simulink model "SteadyCam"  (R2015b)
settings: Solver=FixedStepAuto  StartTime=0.0  StopTime=10.0  FixedStep=Ts  RelTol=1e-3
InitFcn:
  | InitSteady;
values from neighbouring files (symbols this model uses):
  GainGyro = 90/12000    (= 0.0075)    [InitSteady.m]
  InitTime = 2.9    [InitSteady.m]
  PID_Activator = 35    [InitSteady.m]
  Rad2Deg = 180/pi    (= 57.2957795131)    [InitSteady.m]
  Ts = 0.03    [InitSteady.m]
undefined symbols (not defined in the file or in its folder): DiscIntNeverNeededParam, HighValFilter, LowFilterVal
libraries: simulink x3, RASPlib x2
settings Model: Creator=Simón  LastModifiedBy=Simón

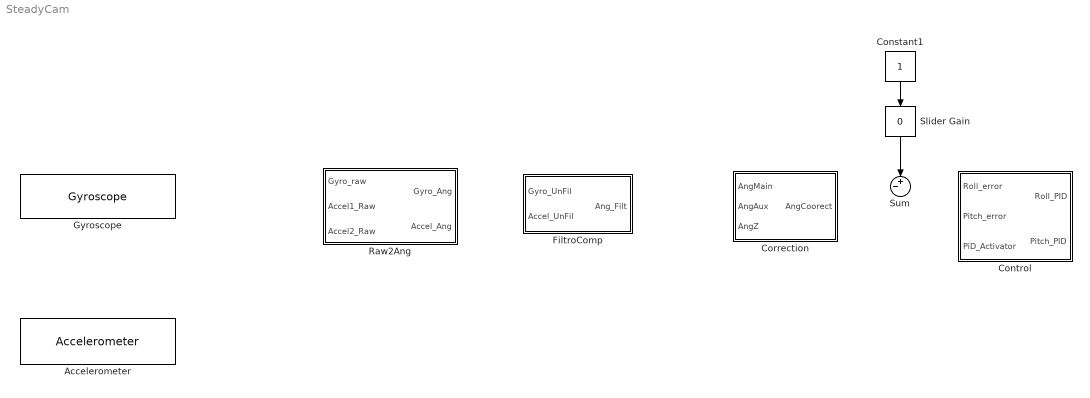
== system SteadyCam ==
  Accelerometer : RASPlib/Accelerometer  SimulateUsing=Code generation
  Constant1 : Constant
  Control : Subsystem
  Correction : Subsystem
  FiltroComp : Subsystem
  Gyroscope : RASPlib/Gyroscope  DLPFmode=0
  Raw2Ang : Subsystem
  Slider Gain : simulink/Math Operations/Slider Gain  low=-25  gain=0  high=35
  Sum : Sum  Inputs=+-|
  wires:
  Constant1/1 -> Slider Gain/1
  Slider Gain/1 -> Sum/1

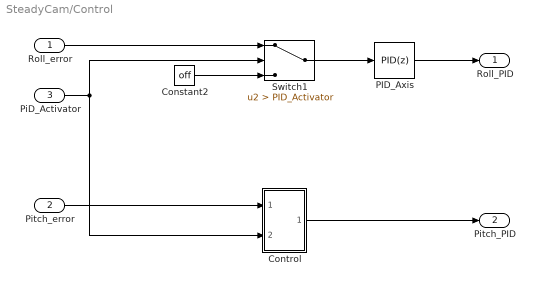
== system SteadyCam/Control ==
  Roll_error : Inport
  Pitch_error : Inport  Port=2
  PiD_Activator : Inport  Port=3
  Constant2 : Constant  Value=off
  Control : Subsystem
  PID_Axis : simulink/Continuous/PID Controller  Controller=PID  TimeDomain=Discrete-time  SampleTime=-1  IntegratorMethod=Forward Euler  FilterMethod=Forward Euler  Form=Parallel  UseFilter=off  ControllerParametersSource=internal  P=0.51  I=0.425  D=0.106  N=30  InitialConditionSource=internal  InitialConditionForIntegrator=0  InitialConditionForFilter=0  ExternalReset=none  LimitOutput=off  UpperSaturationLimit=inf  LowerSaturationLimit=-inf  LinearizeAsGain=off  AntiWindupMode=none  Kb=1  TrackingMode=off  Kt=1  PParamMin=[]  PParamMax=[]  IParamMin=[]  IParamMax=[]  DParamMin=[]  DParamMax=[]  NParamMin=[]  NParamMax=[]  KbParamMin=[]  KbParamMax=[]  KtParamMin=[]  KtParamMax=[]  POutMin=[]  POutMax=[]  IOutMin=[]  IOutMax=[]  DOutMin=[]  DOutMax=[]  NOutMin=[]  NOutMax=[]  KbOutMin=[]  KbOutMax=[]  KtOutMin=[]  KtOutMax=[]  IntegratorOutMin=[]  IntegratorOutMax=[]  FilterOutMin=[]  FilterOutMax=[]  SumOutMin=[]  SumOutMax=[]  SumI1OutMin=[]  SumI1OutMax=[]  SumI2OutMin=[]  SumI2OutMax=[]  SumI3OutMin=[]  SumI3OutMax=[]  SumDOutMin=[]  SumDOutMax=[]  SaturationOutMin=[]  SaturationOutMax=[]  IntegratorContinuousStateAttributes=''  IntegratorStateMustResolveToSignalObject=off  IntegratorRTWStateStorageClass=Auto  FilterContinuousStateAttributes=''  FilterStateMustResolveToSignalObject=off  FilterRTWStateStorageClass=Auto  DifferentiatorICPrevScaledInput=0  DifferentiatorOutMin=[]  DifferentiatorOutMax=[]
  Switch1 : Switch  Criteria=u2 > Threshold  Threshold=PID_Activator
  Roll_PID : Outport
  Pitch_PID : Outport  Port=2
  wires:
  Pitch_error/1 -> Control/1(In1)
  Control/1(Out1) -> Pitch_PID/1
  PID_Axis/1 -> Roll_PID/1
  Switch1/1 -> PID_Axis/1
  PiD_Activator/1 -> Switch1/2, Control/2(Threshold)
  Constant2/1 -> Switch1/3
  Roll_error/1 -> Switch1/1

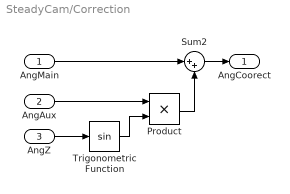
== system SteadyCam/Correction ==
  AngMain : Inport
  AngAux : Inport  Port=2
  AngZ : Inport  Port=3
  Product : Product
  Sum2 : Sum  Inputs=|++
  Trigonometric Function : Trigonometry
  AngCoorect : Outport
  wires:
  AngAux/1 -> Product/1
  Sum2/1 -> AngCoorect/1
  AngZ/1 -> Trigonometric Function/1
  AngMain/1 -> Sum2/1
  Product/1 -> Sum2/2
  Trigonometric Function/1 -> Product/2

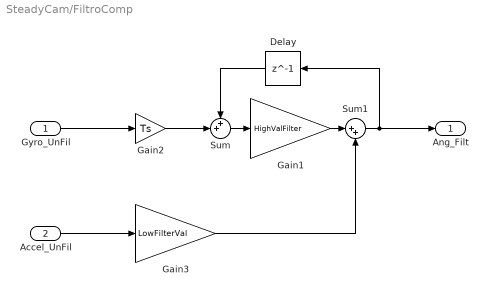
== system SteadyCam/FiltroComp ==
  Gyro_UnFil : Inport
  Accel_UnFil : Inport  Port=2
  Delay : Delay  DelayLength=1  InitialCondition=0
  Gain1 : Gain  Gain=HighValFilter
  Gain2 : Gain  Gain=Ts
  Gain3 : Gain  Gain=LowFilterVal
  Sum : Sum  Inputs=++|
  Sum1 : Sum  Inputs=|++
  Ang_Filt : Outport
  wires:
  Gain3/1 -> Sum1/2
  Gyro_UnFil/1 -> Gain2/1
  Sum1/1 -> Ang_Filt/1, Delay/1
  Gain1/1 -> Sum1/1
  Accel_UnFil/1 -> Gain3/1
  Sum/1 -> Gain1/1
  Delay/1 -> Sum/1
  Gain2/1 -> Sum/2

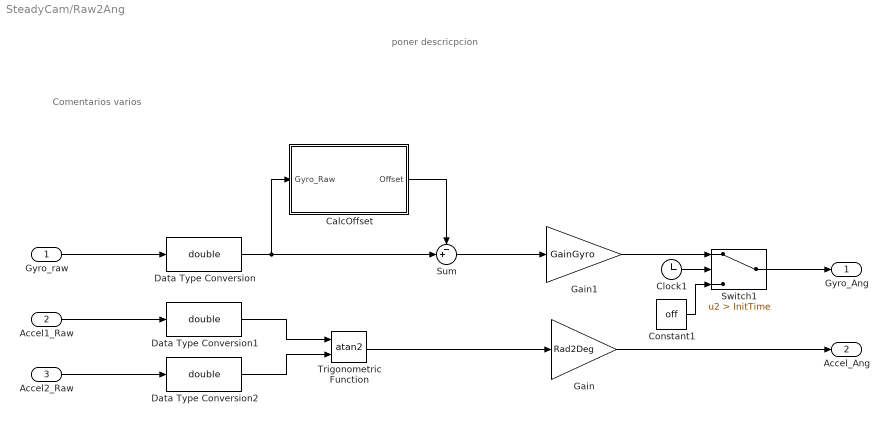
== system SteadyCam/Raw2Ang ==
  note: poner descricpcion
  note: Comentarios varios
  Gyro_raw : Inport
  Accel1_Raw : Inport  Port=2
  Accel2_Raw : Inport  Port=3
  CalcOffset : Subsystem
  Clock1 : Clock
  Constant1 : Constant  Value=off
  Data Type Conversion : DataTypeConversion  OutDataTypeStr=double
  Data Type Conversion1 : DataTypeConversion  OutDataTypeStr=double
  Data Type Conversion2 : DataTypeConversion  OutDataTypeStr=double
  Gain : Gain  Gain=Rad2Deg
  Gain1 : Gain  Gain=GainGyro
  Sum : Sum  Inputs=-+|
  Switch1 : Switch  Criteria=u2 > Threshold  Threshold=InitTime
  Trigonometric Function : Trigonometry  Operator=atan2
  Gyro_Ang : Outport
  Accel_Ang : Outport  Port=2
  wires:
  Accel2_Raw/1 -> Data Type Conversion2/1
  Constant1/1 -> Switch1/3
  Gain1/1 -> Switch1/1
  Gyro_raw/1 -> Data Type Conversion/1
  Trigonometric Function/1 -> Gain/1
  Switch1/1 -> Gyro_Ang/1
  Clock1/1 -> Switch1/2
  Data Type Conversion1/1 -> Trigonometric Function/1
  Data Type Conversion2/1 -> Trigonometric Function/2
  Accel1_Raw/1 -> Data Type Conversion1/1
  Gain/1 -> Accel_Ang/1
  Sum/1 -> Gain1/1
  Data Type Conversion/1 -> CalcOffset/1(Gyro_Raw), Sum/2
  CalcOffset/1(Offset) -> Sum/1

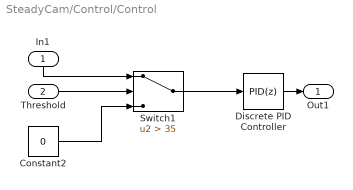
== system SteadyCam/Control/Control ==
  In1 : Inport
  Threshold : Inport  Port=2
  Constant2 : Constant  Value=0
  Discrete PID Controller : simulink/Continuous/PID Controller  Controller=PID  TimeDomain=Discrete-time  SampleTime=-1  IntegratorMethod=Forward Euler  FilterMethod=Forward Euler  Form=Parallel  UseFilter=off  ControllerParametersSource=internal  P=0.51  I=0.425  D=0.106  N=30  InitialConditionSource=internal  InitialConditionForIntegrator=0  InitialConditionForFilter=0  ExternalReset=none  LimitOutput=off  UpperSaturationLimit=inf  LowerSaturationLimit=-inf  LinearizeAsGain=off  AntiWindupMode=none  Kb=1  TrackingMode=off  Kt=1  PParamMin=[]  PParamMax=[]  IParamMin=[]  IParamMax=[]  DParamMin=[]  DParamMax=[]  NParamMin=[]  NParamMax=[]  KbParamMin=[]  KbParamMax=[]  KtParamMin=[]  KtParamMax=[]  POutMin=[]  POutMax=[]  IOutMin=[]  IOutMax=[]  DOutMin=[]  DOutMax=[]  NOutMin=[]  NOutMax=[]  KbOutMin=[]  KbOutMax=[]  KtOutMin=[]  KtOutMax=[]  IntegratorOutMin=[]  IntegratorOutMax=[]  FilterOutMin=[]  FilterOutMax=[]  SumOutMin=[]  SumOutMax=[]  SumI1OutMin=[]  SumI1OutMax=[]  SumI2OutMin=[]  SumI2OutMax=[]  SumI3OutMin=[]  SumI3OutMax=[]  SumDOutMin=[]  SumDOutMax=[]  SaturationOutMin=[]  SaturationOutMax=[]  IntegratorContinuousStateAttributes=''  IntegratorStateMustResolveToSignalObject=off  IntegratorRTWStateStorageClass=Auto  FilterContinuousStateAttributes=''  FilterStateMustResolveToSignalObject=off  FilterRTWStateStorageClass=Auto  DifferentiatorICPrevScaledInput=0  DifferentiatorOutMin=[]  DifferentiatorOutMax=[]
  Switch1 : Switch  Criteria=u2 > Threshold  Threshold=35
  Out1 : Outport
  wires:
  In1/1 -> Switch1/1
  Constant2/1 -> Switch1/3
  Threshold/1 -> Switch1/2
  Switch1/1 -> Discrete PID Controller/1
  Discrete PID Controller/1 -> Out1/1

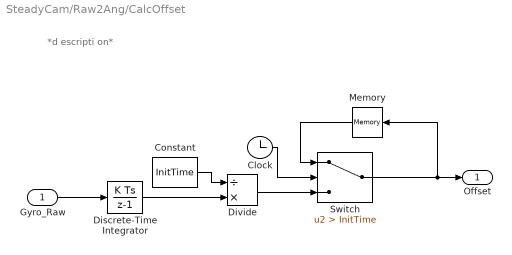
== system SteadyCam/Raw2Ang/CalcOffset ==
  note: *d escripti on*
  Gyro_Raw : Inport
  Clock : Clock
  Constant : Constant  Value=InitTime
  Discrete-Time Integrator : DiscreteIntegrator  InitialConditionSetting=State (most efficient)  SampleTime=Ts  ICPrevOutput=DiscIntNeverNeededParam  ICPrevScaledInput=DiscIntNeverNeededParam
  Divide : Product  Inputs=/*
  Memory : Memory
  Switch : Switch  Criteria=u2 > Threshold  Threshold=InitTime
  Offset : Outport
  wires:
  Divide/1 -> Switch/3
  Discrete-Time Integrator/1 -> Divide/2
  Memory/1 -> Switch/1
  Constant/1 -> Divide/1
  Switch/1 -> Memory/1, Offset/1
  Clock/1 -> Switch/2
  Gyro_Raw/1 -> Discrete-Time Integrator/1
